simulink library "F3M_commonLib"  (R2023b)
settings: Solver=VariableStepAuto  StartTime=0.0  StopTime=10.0  RelTol=1e-3
undefined symbols (not defined in the file): entity, F3_getArrayPos, F3_getLossFilter, F3_ptableToArray, F3_ptableToGain, getIsoVec, isoelestring, m, n, Periodicity, pulsewidth, readAttrib, ressize, updateCurrentEProperties, updateInv
libraries: $bdroot x5
(part 1 of 2)
settings Model: Creator=nshoman  LastModifiedBy=nshoman

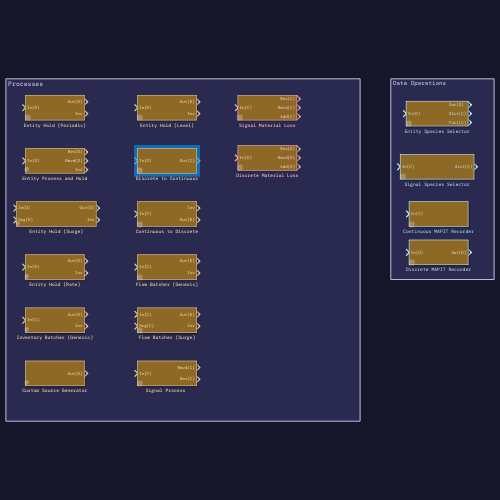
[thumbnail: Simulink's stored preview of the top-level diagram]
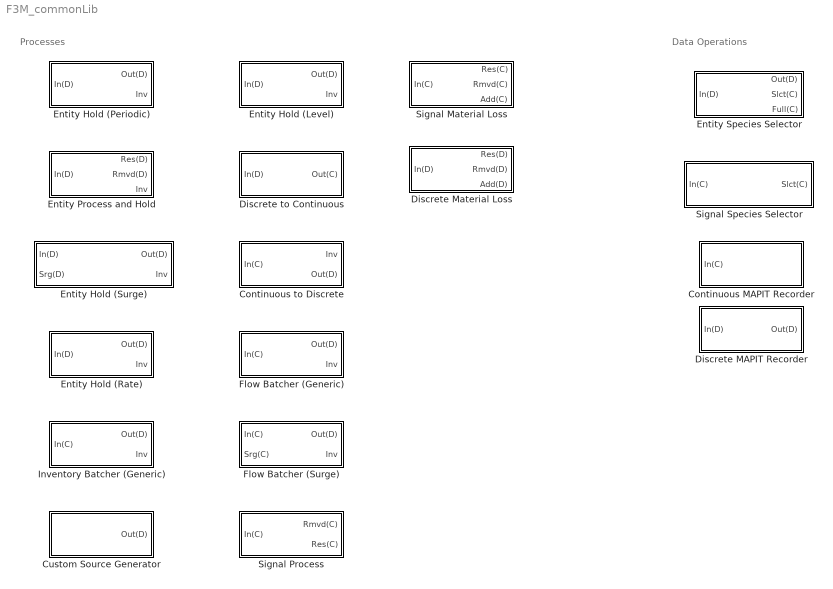
== system F3M_commonLib ==
  note: Processes
  note: Data Operations
  Continuous MAPIT Recorder : Subsystem  mask(Continuous MAPIT Recorder){wsname=simout1}
      mask prompts: wsname "Output variable name"
      mask help: F3M has been designed to work with MAPIT for downstream safeguards analyses. For a traditional material balance evaluation, flows must be integrated over the material balance period. It is important that data in F3M is collected so that, when integrated, input and output terms for the material balance is correct. Sampling too infrequently compared to the flow signals can result in pulses of material that are not recorded or truncated. However, high sampling rates can create excessively large datasets. This block balances these constraints by recording data with an inherited sample rate equal to the models major step, when the signal is non-zero. If the signal is zero, then information is not recorded
      mask init:
      | wsn = get_param(gcb,'wsname');
      |     set_param([gcb,'/TSS/MAPIT_OUT'],'VariableName',wsn);
      mask TypeOptions wsname: simout1
  Continuous to Discrete : Subsystem  mask(Continuous to Discrete){isoelestring=h, pulsewidth=1, size=10, ressize=0}
      mask prompts: isoelestring "Element or isotope (ex: h, u238)"; pulsewidth "Inventory pulse width (hr)"; size "Batch threshold (kg)"; ressize "Residual size (kg)"
      mask help: The continuous to discrete block converts a continuous Simulink signal into a discrete entity.
      mask TypeOptions isoelestring: h
  Custom Source Generator : Subsystem  mask(Custom Source Generator){size=10, period=5, ptable={'h3','1'}}
      mask prompts: size "Item size (kg)"; period "Item period (hr)"; ptable "Source specification table"
      mask help: The custom source generator is a template block for creating entity sources in F3M. The user must either define a source through the mask dialog options or create a function to do so. This block expects that sources will be specified in terms of weight percent expressed as a decimal. The block generates an entitiy with two different attributes, isovec and auxparams.
      mask DialogControl add_entry Prompt: Add entry
      mask DialogControl add_entry Callback:
      | maskObj = Simulink.Mask.get(gcb);
      |     tableControl = maskObj.getDialogControl('ptable');
      |     tableControl.addRow('a','b')
      mask DialogControl remove_entry Prompt: Remove entry
      mask DialogControl remove_entry Callback:
      | maskObj = Simulink.Mask.get(gcb);
      |     tableControl = maskObj.getDialogControl('ptable');
      |     nrow = tableControl.getNumberOfRows();
      |     if nrow>0
      |         tableControl.removeRow(nrow);
      |     end
  Discrete MAPIT Recorder : Subsystem  mask(Discrete MAPIT Recorder){InString=h, wsname=simout1}
      mask prompts: InString "Element or isotope (ex: h, u238)"; wsname "Output variable name"
      mask help: F3M has been designed to work with MAPIT for downstream safeguards analyses. For a traditional material balance evaluation, flows must be integrated over the material balance period. It is important that data in F3M is collected so that, when integrated, input and output terms for the material balance is correct. Discrete items simply output their entity attribute value when present, which eliminates the need for internal logic regarding sample frequency and searching for non-zero signals.
      mask init:
      | wsn = get_param(gcb,'wsname');
      |     set_param([gcb,'/TSS/MAPIT_OUT'],'VariableName',wsn);
      |     set_param([gcb,'/TSS1/MAPIT_OUT'],'VariableName',wsn);
      | 
      |     isn = get_param(gcb, 'InString');
      |     if strcmp(isn, 'all')
      |         set_param([gcb, '/TSS'], 'Commented', 'on');
      |         set_param([gcb, '/TSS1'], 'Commented', 'off');
      |     else
      |         set_param([gcb, '/TSS'], 'Commented', 'off');
      |         set_param([gcb, '/TSS1'], 'Commented', 'on');
      |     end
      mask TypeOptions InString: h
      mask TypeOptions wsname: simout1
  Discrete Material Loss : Subsystem  mask(Entity Material Loss){tStart=0, tEnd=0, lossFrac=0, lossOverride=off, lossOverrideTab={}, replaceBool=off, replaceTable={}}
      mask prompts: tStart "Start time (hr)"; tEnd "End time (hr)"; lossFrac "Removal fraction"; lossOverride "Loss species override"; replaceBool "Replacement material"
      mask help: The entity material loss block is designed to simulate loss, and optionally partial simultaneous replacement, of entities that enter the block. By default, the block removes a fraction of the entities entering the block during the specified interval. This behavior can be modified via the loss species override table wherein fractions can be set for individual elements or isotopes. A replacement table is available to specify replace lost material with a specified element or isotope with a certain fraction.
      mask init:
      | set_param(gcb,'MaskEnables',{'on';'on';'on';'on';'on';'on';'on'})
      |     maskObj = Simulink.Mask.get(gcb); 
      |     btnControl = maskObj.getDialogControl('addSub');
      |     btnControl.Enabled = "off";
      |     btnControl = maskObj.getDialogControl('removeSub');
      |     btnControl.Enabled = "off";
      |     btnControl = maskObj.getDialogControl('addLO');
      |     btnControl.Enabled = "off";
      |     btnControl = maskObj.getDialogControl('removeLO');
      |     btnControl.Enabled = "off";
      mask Callback lossOverride:
      | maskStr = get_param(gcb,'lossOverride');
      |     maskObj = Simulink.Mask.get(gcb);
      |     if strcmp(maskStr,'off')
      |        F = get_param(gcb,'MaskEnables');
      |        F{5} = 'off';
      |        set_param(gcb,'MaskEnables',F);
      |        btnControl = maskObj.getDialogControl('addLO');
      |        btnControl.Enabled = "off";
      |        btnControl = maskObj.getDialogControl('removeLO');
      |        btnControl.Enabled = "off";
      |     else
      |        F = get_param(gcb,'MaskEnables');
      |        F{5} = 'on';
      |        set_param(gcb,'MaskEnables',F);
      |        btnControl = maskObj.getDialogControl('addLO');
      |        btnControl.Enabled = "on";
      |        btnControl = maskObj.getDialogControl('removeLO');
      |        btnControl.Enabled = "on";
      |     end
      mask Callback replaceBool:
      | maskStr = get_param(gcb,'replaceBool');
      |     maskObj = Simulink.Mask.get(gcb);
      |     if strcmp(maskStr,'off')
      |        F = get_param(gcb,'MaskEnables');
      |        F{7} = 'off';
      |        set_param(gcb,'MaskEnables',F);
      |        btnControl = maskObj.getDialogControl('addSub');
      |        btnControl.Enabled = "off";
      |        btnControl = maskObj.getDialogControl('removeSub');
      |        btnControl.Enabled = "off";
      |     else
      |        F = get_param(gcb,'MaskEnables');
      |        F{7} = 'on';
      |        set_param(gcb,'MaskEnables',F);
      |        btnControl = maskObj.getDialogControl('addSub');
      |        btnControl.Enabled = "on";
      |        btnControl = maskObj.getDialogControl('removeSub');
      |        btnControl.Enabled = "on";
      |     end
      mask DialogControl addLO Prompt: Add
      mask DialogControl addLO Callback:
      | maskObj = Simulink.Mask.get(gcb);
      |     tableControl = maskObj.getDialogControl('lossOverrideTab');
      |     tableControl.addRow('a','b')
      mask DialogControl removeLO Prompt: Remove
      mask DialogControl removeLO Callback:
      | maskObj = Simulink.Mask.get(gcb);
      |     tableControl = maskObj.getDialogControl('lossOverrideTab');
      |     nrow = tableControl.getNumberOfRows();
      |     if nrow>0
      |         tableControl.removeRow(nrow);
      |     end
      mask DialogControl addSub Prompt: Add
      mask DialogControl addSub Callback:
      | maskObj = Simulink.Mask.get(gcb);
      |     tableControl = maskObj.getDialogControl('replaceTable');
      |     tableControl.addRow('a','b')
      mask DialogControl removeSub Prompt: Remove
      mask DialogControl removeSub Callback:
      | maskObj = Simulink.Mask.get(gcb);
      |     tableControl = maskObj.getDialogControl('replaceTable');
      |     nrow = tableControl.getNumberOfRows();
      |     if nrow>0
      |         tableControl.removeRow(nrow);
      |     end
  Discrete to Continuous : Subsystem  mask(Discrete to Continuous){width=eps}
      mask prompts: width "Pulse width"
      mask help: The discrete to continuous block converts a discrete entity into a continuous Simulink signal. The discrete item is represented by a square pulse with a width specified by the user. F3M will automatically scale the signal height such that the signal will integrate to the same elemental and isotopic values as the original entity.
      mask init:
      | mask_parameters = Simulink.Mask.get(gcb);
      | width_value = '';
      | for i = 1:length(mask_parameters.Parameters)
      |     if strcmp(mask_parameters.Parameters(i).Name, 'width')
      |         width_value = mask_parameters.Parameters(i).Value;
      |         break;
      |     end
      | end    
      | if strcmp(width_value, "eps")
      |     %width_internal = str2double(get_param(bdroot(),'MaxStep'));
      |     width_internal= 0.05;
      | else
      |     width_internal = str2double(width_value);
      | end
      mask Callback width:
      | mask_parameters = Simulink.Mask.get(gcb);
      | width_value = '';
      | for i = 1:length(mask_parameters.Parameters)
      |     if strcmp(mask_parameters.Parameters(i).Name, 'width')
      |         width_value = mask_parameters.Parameters(i).Value;
      |         break;
      |     end
      | end
      | if strcmp(width_value, "eps")
      |         %width_internal = str2double(get_param(bdroot(),'MaxStep'));
      |         width_internal = 0.05;
      | else
      |     width_internal = str2double(width_value);
      | end
  Entity Hold (Level) : Subsystem  mask(Entity Hold (Level)){nitems=0, time=0}
      mask prompts: nitems "Hold level (items)"; time "Process time (hr)"
      mask help: The entity hold (level) block simply holds a entities at a set level in a queue. If there are more items in queue than the level set point, then entities can leave the queue. The internal queue uses a First In First Out (FIFO) scheme. An optional process time is available which applies a time delay to an entity after it leaves the queue. This parameter can control how quickly entities are able to leave after the level set point has been reached. A continuous inventory term is updated whenever entities enter or leave the block.
  Entity Hold (Periodic) : Subsystem  mask(Entity Process and Hold){t_process=1}
      mask prompts: t_process "Process time (hr)"
      mask help: The entity hold (periodic) block simply holds an discrete entity for a period of time before releasing. The internal queue uses a First In First Out (FIFO) scheme. A continuous inventory term is updated whenever entities enter or leave the block.
  Entity Hold (Rate) : Subsystem  mask(Entity Hold (Rate)){rate=1}
      mask prompts: rate "Rate (item/hr)"
      mask help: This entity hold (rate) block simply holds a discrete entity in a queue. Entities are released at regular rate specified by the mask dialog parameters.
  Entity Hold (Surge) : Subsystem  mask(Entity Hold (Surge)){t_process=1}
      mask prompts: t_process "Process time"
      mask help: The entity hold (surge) block places input entities into a queue with a First In First Out (FIFO) scheme. Entities are only released when a surge signal is received.
  Entity Process and Hold : Subsystem  mask(Entity Process and Hold){t_process=1, ptable={'h3','0.10'}}
      mask prompts: t_process "Process time (hr)"
      mask help: The entity process and hold block holds a discrete entity for a period of time before releasing. If reduction multipliers are specified, then the entity is changed according to the reduction multipliers after any hold period has elapsed. The internal queue uses a First In First Out (FIFO) scheme. A continuous inventory term is updated when entities leave the queue.
      mask DialogControl addRowBtn Prompt: Add Entry
      mask DialogControl addRowBtn Callback:
      | maskObj = Simulink.Mask.get(gcb);
      |     tableControl = maskObj.getDialogControl('ptable');
      |     tableControl.addRow('a','b')
      mask DialogControl removeRowBtn Prompt: Remove Entry
      mask DialogControl removeRowBtn Callback:
      | maskObj = Simulink.Mask.get(gcb);
      |     tableControl = maskObj.getDialogControl('ptable');
      |     nrow = tableControl.getNumberOfRows();
      |     if nrow>0
      |         tableControl.removeRow(nrow);
      |     end
  Entity Species Selector : Subsystem  mask(Entity Species Selector){InString=h, width=0.10}
      mask prompts: InString "Element or isotope (ex: h, u238)"; width "Pulse width"
      mask help: The entity species selector extracts the specified isotope or element attributes of an entity (multiple if several isotopes for the element are tracked). The full signal is also returned, which can be combined with multiple signal selector blocks for additional species-specific signals if desired. This is a convenience block to select certain species of interest from the [1677, 1] shaped attribute that F3M uses for most modeling operations.
      mask TypeOptions InString: h
  Flow Batcher (Generic) : Subsystem  mask(Flow Batcher (Generic)){p1=h, p2=1, p3=0, p4=0}
      mask prompts: p1 "Batch basis (ex: h, u238)"; p2 "Inventory pulse width (hr)"; p3 "Output target size (kg)"; p4 "Residual size (kg)"
      mask help: The generic flow batcher creates discrete entities from an input flow according to user defined settings in the dialog (i.e., creates a batch). The generic flow batcher uses an isotope or element (or other keyword, see overview page) combined with a target size to create an entity.
      mask TypeOptions p1: h
  Flow Batcher (Surge) : Subsystem  mask(Flow Batcher (Surge)){isoelestring=h1, pulsewidth=0, size=0, ressize=0}
      mask prompts: isoelestring "Element or isotope (ex: h, u238)"; pulsewidth "Pulse width (hr)"; size "Output target size (kg)"; ressize "Residual size (kg)"
      mask help: The surge flow batcher creates discrete entities from an input flow according to user defined settings in the dialog (i.e., creates a batch). The surge flow batcher uses an isotope or element (or other keyword, see overview page) combined with a target size to create an entity when a surge signal is supplied.
      mask TypeOptions isoelestring: h1
  Inventory Batcher (Generic) : Subsystem  mask(Inventory Batcher (Generic)){p1=h, p2=1, p3=0, p4=0}
      mask prompts: p1 "Batch basis (ex: h, u238)"; p2 "Inventory pulse width (hr)"; p3 "Output target size (kg)"; p4 "Residual size (kg)"
      mask help: The generic inventory batcher creates discrete entities from an input flow according to user defined settings in the dialog (i.e., creates a batch). This block is similar to the generic flow batcher with the key difference that this block will not output while flow is entering. It is designed to be used with inventories, rather than flows, and expects that there will be periodic, rather than continuous, additions to the inventory will be made.
      mask TypeOptions p1: h
  Signal Material Loss : Subsystem  mask(Signal Material Loss){tStart=0, tEnd=0, lossFrac=0, lossOverride=off, lossOverrideTab={}, replaceBool=off, replaceTable={}}
      mask prompts: tStart "Start time (hr)"; tEnd "End time (hr)"; lossFrac "Removal fraction"; lossOverride "Loss species override"; replaceBool "Replacement material"
      mask help: The signal material loss block is designed to simulate material loss, and optionally simultaneous replacement, of material stream represented by a signal. By default, the block removes a fraction of the signal for the specified amount of time. This behavior can be modified via the loss species override table wherein fractions can be set for individual elements or isotopes. A replacement table is available to specify replace lost material with a specified element or isotope with a certain fraction.
      mask init:
      | set_param(gcb,'MaskEnables',{'on';'on';'on';'on';'on';'on';'on'})
      |     maskObj = Simulink.Mask.get(gcb); 
      |     btnControl = maskObj.getDialogControl('addSub');
      |     btnControl.Enabled = "off";
      |     btnControl = maskObj.getDialogControl('removeSub');
      |     btnControl.Enabled = "off";
      |     btnControl = maskObj.getDialogControl('addLO');
      |     btnControl.Enabled = "off";
      |     btnControl = maskObj.getDialogControl('removeLO');
      |     btnControl.Enabled = "off";
      mask Callback lossOverride:
      | maskStr = get_param(gcb,'lossOverride');
      |     maskObj = Simulink.Mask.get(gcb);
      |     if strcmp(maskStr,'off')
      |        F = get_param(gcb,'MaskEnables');
      |        F{5} = 'off';
      |        set_param(gcb,'MaskEnables',F);
      |        btnControl = maskObj.getDialogControl('addLO');
      |        btnControl.Enabled = "off";
      |        btnControl = maskObj.getDialogControl('removeLO');
      |        btnControl.Enabled = "off";
      |     else
      |        F = get_param(gcb,'MaskEnables');
      |        F{5} = 'on';
      |        set_param(gcb,'MaskEnables',F);
      |        btnControl = maskObj.getDialogControl('addLO');
      |        btnControl.Enabled = "on";
      |        btnControl = maskObj.getDialogControl('removeLO');
      |        btnControl.Enabled = "on";
      |     end
      mask Callback replaceBool:
      | maskStr = get_param(gcb,'replaceBool');
      |     maskObj = Simulink.Mask.get(gcb);
      |     if strcmp(maskStr,'off')
      |        F = get_param(gcb,'MaskEnables');
      |        F{7} = 'off';
      |        set_param(gcb,'MaskEnables',F);
      |        btnControl = maskObj.getDialogControl('addSub');
      |        btnControl.Enabled = "off";
      |        btnControl = maskObj.getDialogControl('removeSub');
      |        btnControl.Enabled = "off";
      |     else
      |        F = get_param(gcb,'MaskEnables');
      |        F{7} = 'on';
      |        set_param(gcb,'MaskEnables',F);
      |        btnControl = maskObj.getDialogControl('addSub');
      |        btnControl.Enabled = "on";
      |        btnControl = maskObj.getDialogControl('removeSub');
      |        btnControl.Enabled = "on";
      |     end
      mask DialogControl addLO Prompt: Add
      mask DialogControl addLO Callback:
      | maskObj = Simulink.Mask.get(gcb);
      |     tableControl = maskObj.getDialogControl('lossOverrideTab');
      |     tableControl.addRow('a','b')
      mask DialogControl removeLO Prompt: Remove
      mask DialogControl removeLO Callback:
      | maskObj = Simulink.Mask.get(gcb);
      |     tableControl = maskObj.getDialogControl('lossOverrideTab');
      |     nrow = tableControl.getNumberOfRows();
      |     if nrow>0
      |         tableControl.removeRow(nrow);
      |     end
      mask DialogControl addSub Prompt: Add
      mask DialogControl addSub Callback:
      | maskObj = Simulink.Mask.get(gcb);
      |     tableControl = maskObj.getDialogControl('replaceTable');
      |     tableControl.addRow('a','b')
      mask DialogControl removeSub Prompt: Remove
      mask DialogControl removeSub Callback:
      | maskObj = Simulink.Mask.get(gcb);
      |     tableControl = maskObj.getDialogControl('replaceTable');
      |     nrow = tableControl.getNumberOfRows();
      |     if nrow>0
      |         tableControl.removeRow(nrow);
      |     end
  "Signal Process " : Subsystem  mask(Signal Process){ptable={}}
      mask help: The signal process block applies user specified modification fractions to the signal to simulate a process. These values are assumed to be in [0,1], although any float can be provided.
      mask DialogControl addRowBtn Prompt: Add Entry
      mask DialogControl addRowBtn Callback:
      | maskObj = Simulink.Mask.get(gcb);
      |     tableControl = maskObj.getDialogControl('ptable');
      |     tableControl.addRow('a','b')
      mask DialogControl removeRowBtn Prompt: Remove Entry
      mask DialogControl removeRowBtn Callback:
      | maskObj = Simulink.Mask.get(gcb);
      |     tableControl = maskObj.getDialogControl('ptable');
      |     nrow = tableControl.getNumberOfRows();
      |     if nrow>0
      |         tableControl.removeRow(nrow);
      |     end
  Signal Species Selector : Subsystem  mask(Signal Species Selector){InString=h}
      mask prompts: InString "Element or isotope (ex: h, u238)"
      mask help: The signal species selector extracts the specified isotope signal or element signal (multiple if several isotopes for the element are tracked). This is a convenience block to select certain species of interest from the [1677, 1] shaped signal that F3M uses for most modeling operations.
      mask TypeOptions InString: h

== system F3M_commonLib/Continuous MAPIT Recorder ==
  In(C) : Inport
  Constant : Constant
  Constant1 : Constant  Value=0
  Memory : Memory
  Memory1 : Memory
  Memory2 : Memory
  Sum : Sum  Inputs=++++
  Sum of Elements : Sum  Inputs=+
  Switch : Switch  Criteria=u2 ~= 0  SaturateOnIntegerOverflow=off  InputSameDT=off
  TSS : Subsystem  TreatAsAtomicUnit=on
  wires:
  Constant/1 -> Switch/1
  Constant1/1 -> Switch/3
  In(C)/1 -> TSS/1(In(C)), Sum of Elements/1
  Sum of Elements/1 -> Switch/2
  Switch/1 -> Sum/1, Memory/1
  Memory/1 -> Sum/2, Memory1/1
  Memory1/1 -> Sum/3, Memory2/1
  Sum/1 -> TSS/Enable
  Memory2/1 -> Sum/4

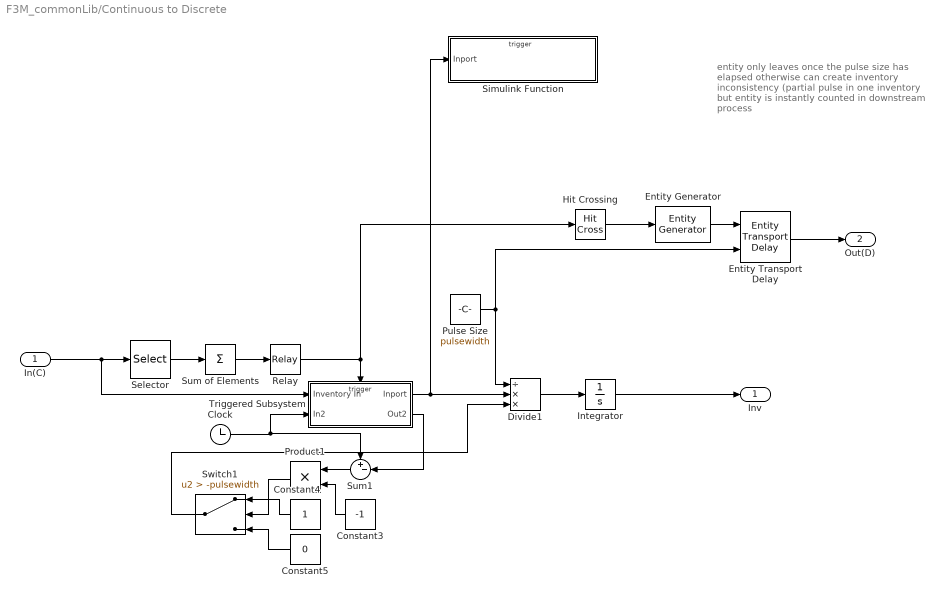
== system F3M_commonLib/Continuous to Discrete ==
  note: entity only leaves once
      | the pulse size has elapsed
      | otherwise can create inventory
      | inconsistency (partial pulse
      | in one inventory but entity is
      | instantly counted in downstream
      | process
  In(C) : Inport
  Clock : Clock
  Constant3 : Constant  Value=-1
  Constant4 : Constant
  Constant5 : Constant  Value=0
  Divide1 : Product  Inputs=/**
  Entity Transport Delay : EntityTransportDelay  InputPortMessageModes=m,n  OutputPortMessageModes=m
  Entity Generator : EntityGenerator  InputPortMessageModes=m  OutputPortMessageModes=m  GenerationMethod=Event-based  GenerateAction=entity.isovec = updateIsovec();  AttributeName=isovec|auxparam  AttributeInitialValue=zeros(1677,1)|1  EntityType=Structured  EntityTypeName=Entity
      settings: InputPortMap=u0
  Hit Crossing : HitCross  OutputPortMessageModes=m  HitCrossingOffset=1  HitCrossingDirection=rising  HitCrossingOutputType=Message
  Integrator : Integrator
  Product1 : Product
  Pulse Size : Constant  Value=pulsewidth
  Relay : Relay  OnSwitchValue=size  OffSwitchValue=ressize
  Selector : Selector  InputPortWidth=1677  IndexOptions=Index vector (dialog)  Indices=F3_getArrayPos(isoelestring)  OutputSizes=1
  Simulink Function : Subsystem  TreatAsAtomicUnit=on
  Sum of Elements : Sum  Inputs=+
  Sum1 : Sum  Inputs=+-|
  Switch1 : Switch  Criteria=u2 > Threshold  Threshold=-pulsewidth  SaturateOnIntegerOverflow=off  InputSameDT=off
      settings: AttributesFormatString=-pulseSize
  Triggered Subsystem : Subsystem  TreatAsAtomicUnit=on
  Inv : Outport
  Out(D) : Outport  Port=2
  wires:
  Integrator/1 -> Inv/1
  Clock/1 -> Sum1/1, Triggered Subsystem/2(In2)
  Constant5/1 -> Switch1/3
  Sum of Elements/1 -> Relay/1
  Constant3/1 -> Product1/2
  Relay/1 -> Hit Crossing/1, Triggered Subsystem/Trigger
  Triggered Subsystem/2(Out2) -> Sum1/2
  Divide1/1 -> Integrator/1
  Switch1/1 -> Divide1/3
  Triggered Subsystem/1(Inport) -> Divide1/2, Simulink Function/1(Inport)
  In(C)/1 -> Triggered Subsystem/1(Inventory In), Selector/1
  Product1/1 -> Switch1/2
  Constant4/1 -> Switch1/1
  Sum1/1 -> Product1/1
  Selector/1 -> Sum of Elements/1
  Hit Crossing/1 -> Entity Generator/1
  Entity Generator/1 -> Entity Transport Delay/1
  Entity Transport Delay/1 -> Out(D)/1
  Pulse Size/1 -> Entity Transport Delay/2, Divide1/1

== system F3M_commonLib/Custom Source Generator ==
  Entity Generator : EntityGenerator  OutputPortMessageModes=m  Period=period  GenerateAction=entity.isovec = getInitialIsos();  AttributeName=isovec|auxparam  AttributeInitialValue=zeros(1677,1)|1  EntityType=Structured  EntityTypeName=Entity
  Simulink Function : Subsystem  TreatAsAtomicUnit=on
  Out(D) : Outport
  wires:
  Entity Generator/1 -> Out(D)/1

== system F3M_commonLib/Discrete MAPIT Recorder ==
  In(D) : Inport
  Entity Server : EntityServer  InputPortMessageModes=m  OutputPortMessageModes=m  Capacity=1  ServiceTimeValue=0  ExitAction=readAttrib(entity.isovec)
  TSS : Subsystem  TreatAsAtomicUnit=on
  TSS1 : Subsystem  Commented=on  TreatAsAtomicUnit=on
  Out(D) : Outport
  wires:
  In(D)/1 -> Entity Server/1
  Entity Server/1 -> Out(D)/1

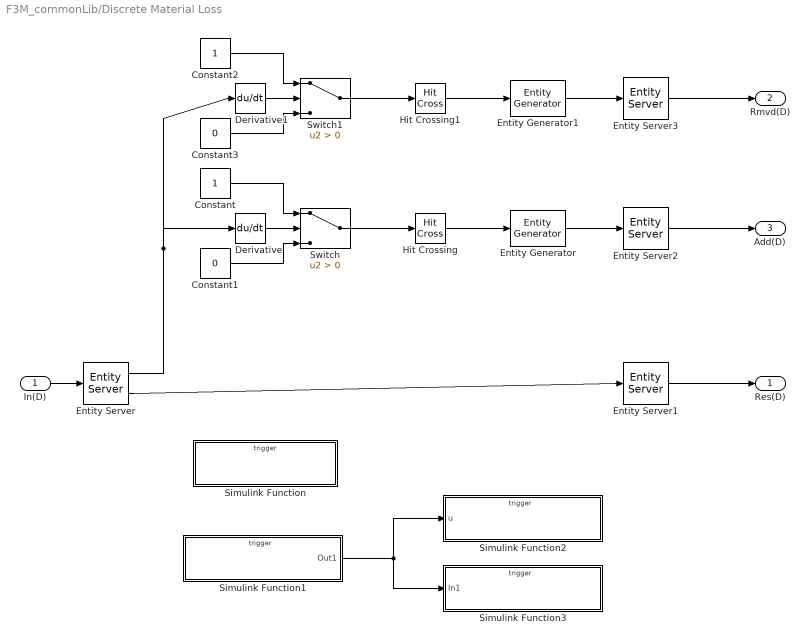
== system F3M_commonLib/Discrete Material Loss ==
  In(D) : Inport
  Constant : Constant
  Constant1 : Constant  Value=0
  Constant2 : Constant
  Constant3 : Constant  Value=0
  Derivative : Derivative
  Derivative1 : Derivative
  Entity Generator : EntityGenerator  InputPortMessageModes=m  OutputPortMessageModes=m  GenerationMethod=Event-based  AttributeName=isovec|auxparam  AttributeInitialValue=zeros(1677,1)|1  EntityType=Structured  EntityTypeName=Entity
      settings: InputPortMap=u0
  Entity Generator1 : EntityGenerator  InputPortMessageModes=m  OutputPortMessageModes=m  GenerationMethod=Event-based  AttributeName=isovec|auxparam  AttributeInitialValue=zeros(1677,1)|1  EntityType=Structured  EntityTypeName=Entity
      settings: InputPortMap=u0
  Entity Server : EntityServer  InputPortMessageModes=m  OutputPortMessageModes=n,m  Capacity=inf  ServiceTimeValue=0  EntryAction=updateCurrentEProperties(entity.isovec);  NumberEntitiesDeparted=on
      settings: OutputPortMap=o0,o9
  Entity Server1 : EntityServer  InputPortMessageModes=m  OutputPortMessageModes=m  Capacity=inf  ServiceTimeValue=0  ServiceCompleteAction=entity.isovec = applyAllFilters(entity.isovec);
  Entity Server2 : EntityServer  InputPortMessageModes=m  OutputPortMessageModes=m  Capacity=inf  ServiceTimeValue=0  ServiceCompleteAction=entity.isovec=applyGainFilterGainE();
  Entity Server3 : EntityServer  InputPortMessageModes=m  OutputPortMessageModes=m  Capacity=inf  ServiceTimeValue=0  ServiceCompleteAction=entity.isovec=applyLossFilterLossE();
  Hit Crossing : HitCross  HitCrossingDirection=rising  HitCrossingOutputType=Message
  Hit Crossing1 : HitCross  HitCrossingDirection=rising  HitCrossingOutputType=Message
  Simulink Function : Subsystem  TreatAsAtomicUnit=on
  Simulink Function1 : Subsystem  TreatAsAtomicUnit=on
  Simulink Function2 : Subsystem  TreatAsAtomicUnit=on
  Simulink Function3 : Subsystem  TreatAsAtomicUnit=on
  Switch : Switch  Criteria=u2 > Threshold  SaturateOnIntegerOverflow=off  InputSameDT=off
  Switch1 : Switch  Criteria=u2 > Threshold  SaturateOnIntegerOverflow=off  InputSameDT=off
  Res(D) : Outport
  Rmvd(D) : Outport  Port=2
  Add(D) : Outport  Port=3
  wires:
  In(D)/1 -> Entity Server/1
  Entity Server/2 -> Entity Server1/1
  Entity Server1/1 -> Res(D)/1
  Derivative/1 -> Switch/2
  Entity Server/1 -> Derivative1/1, Derivative/1
  Constant/1 -> Switch/1
  Constant1/1 -> Switch/3
  Switch/1 -> Hit Crossing/1
  Entity Generator/1 -> Entity Server2/1
  Entity Server2/1 -> Add(D)/1
  Hit Crossing/1 -> Entity Generator/1
  Entity Server3/1 -> Rmvd(D)/1
  Entity Generator1/1 -> Entity Server3/1
  Constant2/1 -> Switch1/1
  Switch1/1 -> Hit Crossing1/1
  Constant3/1 -> Switch1/3
  Hit Crossing1/1 -> Entity Generator1/1
  Derivative1/1 -> Switch1/2
  Simulink Function1/1(Out1) -> Simulink Function3/1(In1), Simulink Function2/1(u)

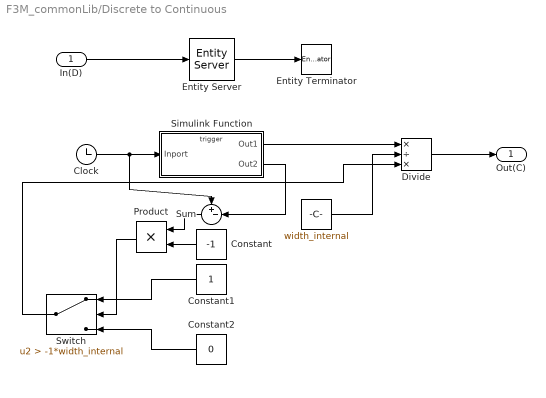
== system F3M_commonLib/Discrete to Continuous ==
  In(D) : Inport
  " " : Constant  Value=width_internal
  Clock : Clock
  Constant : Constant  Value=-1
  Constant1 : Constant
  Constant2 : Constant  Value=0
  Divide : Product  Inputs=*/*
  Entity Server : EntityServer  InputPortMessageModes=m  OutputPortMessageModes=m  Capacity=1  ExitAction=getIsoVec(entity.isovec);
  Entity Terminator : EntityTerminator  InputPortMessageModes=m
  Product : Product
  Simulink Function : Subsystem  TreatAsAtomicUnit=on
  Sum : Sum  Inputs=+-|
  Switch : Switch  Criteria=u2 > Threshold  Threshold=-1*width_internal  SaturateOnIntegerOverflow=off  InputSameDT=off
  Out(C) : Outport
  wires:
  In(D)/1 -> Entity Server/1
  Entity Server/1 -> Entity Terminator/1
  Clock/1 -> Sum/1, Simulink Function/1(Inport)
  Simulink Function/1(Out1) -> Divide/1
  Divide/1 -> Out(C)/1
  Simulink Function/2(Out2) -> Sum/2
  Sum/1 -> Product/1
  Constant/1 -> Product/2
  Constant2/1 -> Switch/3
  Constant1/1 -> Switch/1
  Product/1 -> Switch/2
  Switch/1 -> Divide/3
  " "/1 -> Divide/2

== system F3M_commonLib/Entity Hold (Level) ==
  In(D) : Inport
  Constant : Constant
  Constant1 : Constant  Value=-1
  Entity Gate : EntityGate  InputPortMessageModes=m,m  OutputPortMessageModes=m
  Entity Server : EntityServer  InputPortMessageModes=m  OutputPortMessageModes=n,m  Capacity=inf  ServiceTimeValue=0  EntryAction=updateInv(entity.isovec,1)  NumberEntitiesInBlock=on
      settings: OutputPortMap=o1,o9
  Entity Server1 : EntityServer  InputPortMessageModes=m  OutputPortMessageModes=m  Capacity=1  ServiceTimeValue=time  ExitAction=updateInv(entity.isovec,-1)
  Message Send : Send  OutputPortMessageModes=m
  Simulink Function1 : $bdroot/Entity Hold (Periodic)/Simulink Function  SystemSampleTime=-1  VariantActivationTime=update diagram  AllowFlexibleInterface=on  Latency=0  AutoFrameSizeCalculation=off
      settings: LibrarySourceBlock=sldelib/Simulink Function
  Switch : Switch  Threshold=nitems  SaturateOnIntegerOverflow=off  InputSameDT=off
  Out(D) : Outport
  Inv : Outport  Port=2
  wires:
  Simulink Function1/1 -> Inv/1
  In(D)/1 -> Entity Server/1
  Entity Server/2 -> Entity Gate/2
  Entity Gate/1 -> Entity Server1/1
  Entity Server1/1 -> Out(D)/1
  Entity Server/1 -> Switch/2
  Constant/1 -> Switch/1
  Constant1/1 -> Switch/3
  Switch/1 -> Message Send/1
  Message Send/1 -> Entity Gate/1

== system F3M_commonLib/Entity Hold (Periodic) ==
  "In(D) " : Inport
  Entity Server1 : EntityServer  InputPortMessageModes=m  OutputPortMessageModes=m  Capacity=inf  ServiceTimeValue=t_process  EntryAction=updateInv(entity.isovec,1)  ExitAction=updateInv(entity.isovec,-1)
  Simulink Function : Subsystem  TreatAsAtomicUnit=on
      settings: LibrarySourceBlock=sldelib/Simulink Function
  Out(D) : Outport
  Inv : Outport  Port=2
  wires:
  "In(D) "/1 -> Entity Server1/1
  Entity Server1/1 -> Out(D)/1
  Simulink Function/1(y) -> Inv/1

== system F3M_commonLib/Entity Hold (Rate) ==
  In(D) : Inport
  Entity Server : EntityServer  InputPortMessageModes=m  OutputPortMessageModes=m  Capacity=inf  ServiceTimeValue=1/rate
  Simulink Function : $bdroot/Entity Hold (Periodic)/Simulink Function  SystemSampleTime=-1  VariantActivationTime=update diagram  AllowFlexibleInterface=on  Latency=0  AutoFrameSizeCalculation=off
      settings: LibrarySourceBlock=sldelib/Simulink Function
  Out(D) : Outport
  Inv : Outport  Port=2
  wires:
  In(D)/1 -> Entity Server/1
  Entity Server/1 -> Out(D)/1
  Simulink Function/1 -> Inv/1

== system F3M_commonLib/Entity Hold (Surge) ==
  In(D) : Inport
  Srg(D) : Inport  Port=2
  Entity Gate : EntityGate  InputPortMessageModes=m,m  OutputPortMessageModes=m
  Entity Queue : Queue  InputPortMessageModes=m  OutputPortMessageModes=m  Capacity=inf
  Entity Server : EntityServer  InputPortMessageModes=m  OutputPortMessageModes=m  Capacity=inf  ServiceTimeValue=t_process  EntryAction=updateInv(entity.isovec,1)
  Entity Server1 : EntityServer  InputPortMessageModes=m  OutputPortMessageModes=m  Capacity=inf  ServiceTimeValue=0  ExitAction=updateInv(entity.isovec,-1)
  Simulink Function1 : $bdroot/Entity Hold (Periodic)/Simulink Function  SystemSampleTime=-1  VariantActivationTime=update diagram  AllowFlexibleInterface=on  Latency=0  AutoFrameSizeCalculation=off
      settings: LibrarySourceBlock=sldelib/Simulink Function
  Out(D) : Outport
  Inv : Outport  Port=2
  wires:
  Entity Queue/1 -> Entity Gate/2
  Entity Gate/1 -> Entity Server1/1
  Srg(D)/1 -> Entity Gate/1
  In(D)/1 -> Entity Server/1
  Entity Server/1 -> Entity Queue/1
  Entity Server1/1 -> Out(D)/1
  Simulink Function1/1 -> Inv/1

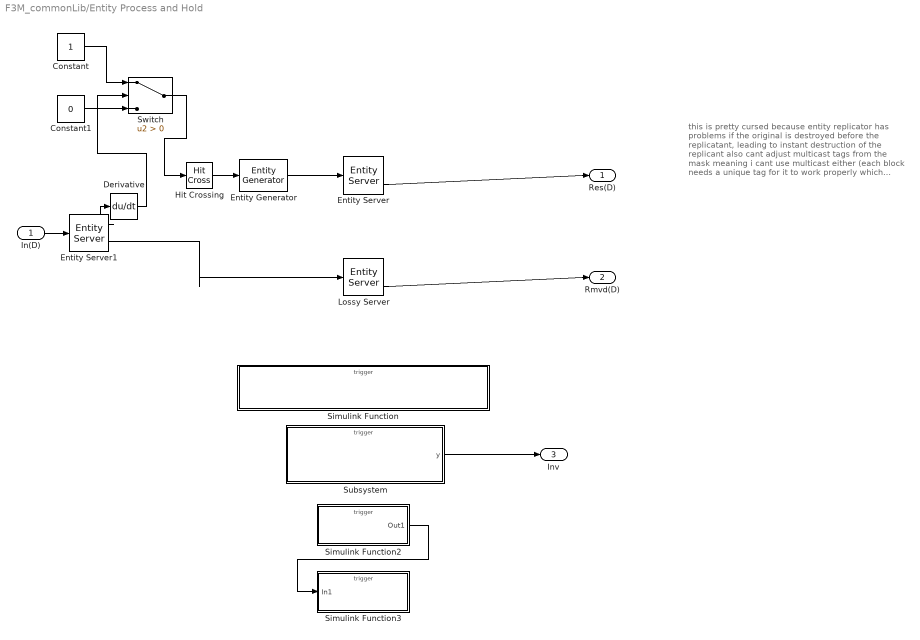
== system F3M_commonLib/Entity Process and Hold ==
  note: this is pretty cursed because
      | entity replicator has problems
      | if the original is destroyed
      | before the replicatant, leading
      | to instant destruction of the
      | replicant
      |
      | also cant adjust multicast tags
      | from the mask meaning i cant
      | use multicast either (each
      | block needs a unique tag
      | for it to work properly which
      | needs to be assigned programatically)
      |
      | the multiple servers ensures
      | things happen in the proper order
  In(D) : Inport
  Constant : Constant
  Constant1 : Constant  Value=0
  Derivative : Derivative
  Entity Generator : EntityGenerator  InputPortMessageModes=m  OutputPortMessageModes=m  GenerationMethod=Event-based  Period=Periodicity  GenerateAction=entity.isovec = getEntityValue();  AttributeName=isovec|auxparam  AttributeInitialValue=zeros(1677,1)|1  EntityType=Structured  EntityTypeName=Entity
      settings: InputPortMap=u0
  Entity Server : EntityServer  InputPortMessageModes=m  OutputPortMessageModes=n,m  Capacity=inf  ServiceTimeValue=t_process  ServiceCompleteAction=entity.isovec=calculateNewEntity(entity.isovec,0);  ExitAction=updateInv(entity.isovec,-1)  NumberEntitiesDeparted=on
      settings: OutputPortMap=o0,o9
  Entity Server1 : EntityServer  InputPortMessageModes=m  OutputPortMessageModes=n,m  Capacity=inf  ServiceTimeValue=0  EntryAction=|  NumberEntitiesDeparted=on
      | updateInv(entity.isovec,1)
      | updateLatestEntity(entity.isovec);
      settings: OutputPortMap=o0,o9
  Hit Crossing : HitCross  OutputPortMessageModes=m  HitCrossingDirection=rising  HitCrossingOutputType=Message
  Lossy Server : EntityServer  InputPortMessageModes=m  OutputPortMessageModes=n,m  Capacity=inf  ServiceTimeValue=t_process  ServiceCompleteAction=entity.isovec=calculateNewEntity(entity.isovec,1);  ExitAction=updateInv(entity.isovec,-1)  NumberEntitiesDeparted=on
      settings: OutputPortMap=o0,o9
  Simulink Function : Subsystem  TreatAsAtomicUnit=on
      settings: LibrarySourceBlock=sldelib/Simulink Function
  Simulink Function2 : Subsystem  TreatAsAtomicUnit=on
  Simulink Function3 : Subsystem  TreatAsAtomicUnit=on
  Subsystem : Subsystem
  Switch : Switch  Criteria=u2 > Threshold  SaturateOnIntegerOverflow=off  InputSameDT=off
  Res(D) : Outport
  Rmvd(D) : Outport  Port=2
  Inv : Outport  Port=3
  wires:
  Hit Crossing/1 -> Entity Generator/1
  Entity Generator/1 -> Entity Server/1
  Lossy Server/2 -> Rmvd(D)/1
  Switch/1 -> Hit Crossing/1
  Entity Server/2 -> Res(D)/1
  Subsystem/1(y) -> Inv/1
  Entity Server1/2 -> Lossy Server/1
  Constant/1 -> Switch/1
  Simulink Function2/1(Out1) -> Simulink Function3/1(In1)
  Entity Server1/1 -> Derivative/1
  Constant1/1 -> Switch/3
  Derivative/1 -> Switch/2
  In(D)/1 -> Entity Server1/1

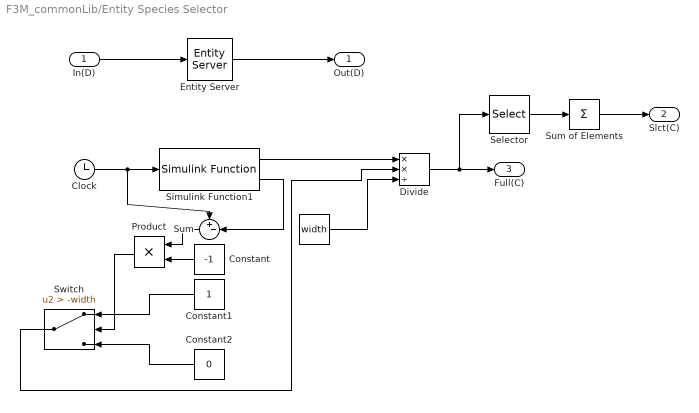
== system F3M_commonLib/Entity Species Selector ==
  In(D) : Inport
  " " : Constant  Value=width
  Clock : Clock
  Constant : Constant  Value=-1
  Constant1 : Constant
  Constant2 : Constant  Value=0
  Divide : Product  Inputs=**/
  Entity Server : EntityServer  InputPortMessageModes=m  OutputPortMessageModes=m  Capacity=inf  ServiceTimeValue=0  ExitAction=getIsoVec(entity.isovec)
  Product : Product
  Selector : Selector  InputPortWidth=1677  IndexOptions=Index vector (dialog)  Indices=F3_getArrayPos(InString)  OutputSizes=1
  Simulink Function1 : $bdroot/Discrete to Continuous/Simulink Function  SystemSampleTime=-1  VariantActivationTime=update diagram  AllowFlexibleInterface=on  Latency=0  AutoFrameSizeCalculation=off
  Sum : Sum  Inputs=+-|
  Sum of Elements : Sum  Inputs=+
  Switch : Switch  Criteria=u2 > Threshold  Threshold=-width  SaturateOnIntegerOverflow=off  InputSameDT=off
  "Out(D) " : Outport
  Slct(C) : Outport  Port=2
  Full(C) : Outport  Port=3
  wires:
  In(D)/1 -> Entity Server/1
  Entity Server/1 -> "Out(D) "/1
  Constant/1 -> Product/2
  Simulink Function1/1 -> Divide/1
  Constant2/1 -> Switch/3
  Sum/1 -> Product/1
  Divide/1 -> Selector/1, Full(C)/1
  Simulink Function1/2 -> Sum/2
  Clock/1 -> Sum/1, Simulink Function1/1
  Product/1 -> Switch/2
  Constant1/1 -> Switch/1
  " "/1 -> Divide/3
  Switch/1 -> Divide/2
  Selector/1 -> Sum of Elements/1
  Sum of Elements/1 -> Slct(C)/1

== system F3M_commonLib/Flow Batcher (Generic) ==
  In(C) : Inport
  "Continuous to Discrete " : Subsystem  Description=requires eval on mask so isn't a direct link of continuous to discrete  mask{isoelestring=p1, pulsewidth=p2, size=p3, ressize=p4}
      mask prompts: isoelestring "Element or isotope (ex: h, u238)"; pulsewidth "Pulse width (hr)"; size "Output target size (kg)"; ressize "Residual size (kg)"
      mask TypeOptions isoelestring: h
  Integrator : Integrator
  Sum : Sum  Inputs=+-
  Out(D) : Outport
  Inv : Outport  Port=2
  wires:
  In(C)/1 -> Integrator/1
  Integrator/1 -> Sum/1
  Sum/1 -> "Continuous to Discrete "/1(Inventory In), Inv/1
  "Continuous to Discrete "/2(Entity) -> Out(D)/1
  "Continuous to Discrete "/1(Inventory Reduce) -> Sum/2

== system F3M_commonLib/Flow Batcher (Surge) ==
  In(C) : Inport
  Srg(C) : Inport  Port=2
  Continuous to Discrete (Surge) : Subsystem  mask{isoelestring=isoelestring, pulsewidth=pulsewidth, size=size, ressize=ressize}
      mask prompts: isoelestring "Element or isotope (ex: h, u238)"; pulsewidth "Pulse width (hr)"; size "Output target size (kg)"; ressize "Residual size (kg)"
      mask TypeOptions isoelestring: isoelestring
  Integrator : Integrator
  Sum : Sum  Inputs=+-
  Out(D) : Outport
  Inv : Outport  Port=2
  wires:
  In(C)/1 -> Integrator/1
  Integrator/1 -> Sum/1
  Sum/1 -> Continuous to Discrete (Surge)/1(Inventory In), Inv/1
  Srg(C)/1 -> Continuous to Discrete (Surge)/2(Surge)
  Continuous to Discrete (Surge)/1(Inventory Reduce) -> Sum/2
  Continuous to Discrete (Surge)/2(Entity) -> Out(D)/1

== system F3M_commonLib/Inventory Batcher (Generic) ==
  In(C) : Inport
  Batcher : Subsystem
  Integrator : Integrator
  Sum : Sum  Inputs=+-
  Out(D) : Outport
  Inv : Outport  Port=2
  wires:
  In(C)/1 -> Integrator/1
  Integrator/1 -> Sum/1
  Sum/1 -> Batcher/1(Inventory In), Inv/1
  Batcher/1(Reduce) -> Sum/2
  Batcher/2(Entity) -> Out(D)/1

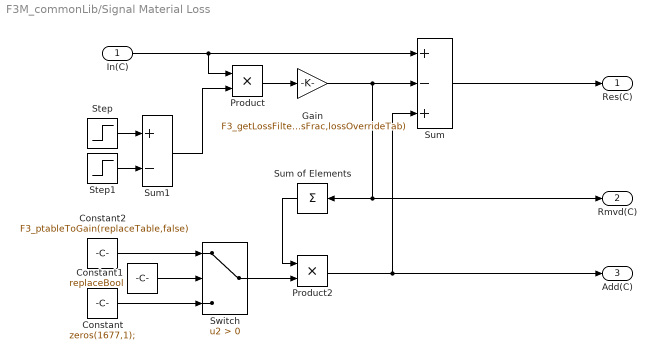
== system F3M_commonLib/Signal Material Loss ==
  In(C) : Inport
  Constant : Constant  Value=zeros(1677,1);
  Constant1 : Constant  Value=replaceBool
  Constant2 : Constant  Value=F3_ptableToGain(replaceTable,false)
  Gain : Gain  Gain=F3_getLossFilter(lossFrac,lossOverrideTab)
  Product : Product
  Product2 : Product
  Step : Step  Time=tStart  SampleTime=0
  Step1 : Step  Time=tEnd  SampleTime=0
  Sum : Sum  Inputs=+-+
  Sum of Elements : Sum  Inputs=+
  Sum1 : Sum  Inputs=+-
  Switch : Switch  Criteria=u2 > Threshold  SaturateOnIntegerOverflow=off  InputSameDT=off
  Res(C) : Outport
  Rmvd(C) : Outport  Port=2
  Add(C) : Outport  Port=3
  wires:
  Sum/1 -> Res(C)/1
  In(C)/1 -> Product/1, Sum/1
  Product/1 -> Gain/1
  Step/1 -> Sum1/1
  Step1/1 -> Sum1/2
  Sum1/1 -> Product/2
  Gain/1 -> Rmvd(C)/1, Sum of Elements/1, Sum/2
  Switch/1 -> Product2/2
  Constant/1 -> Switch/3
  Constant1/1 -> Switch/2
  Constant2/1 -> Switch/1
  Sum of Elements/1 -> Product2/1
  Product2/1 -> Sum/3, Add(C)/1

== system F3M_commonLib/Signal Process  ==
  In(C) : Inport
  Gain : Gain  Gain=F3_ptableToGain(ptable,false)
  Sum : Sum  Inputs=-+|
  Rmvd(C) : Outport
  Res(C) : Outport  Port=2
  wires:
  In(C)/1 -> Sum/2, Gain/1
  Gain/1 -> Rmvd(C)/1, Sum/1
  Sum/1 -> Res(C)/1

== system F3M_commonLib/Signal Species Selector ==
  In(C) : Inport
  Selector : Selector  InputPortWidth=1677  IndexOptions=Index vector (dialog)  Indices=F3_getArrayPos(InString)  OutputSizes=1
  Sum of Elements : Sum  Inputs=+
  Slct(C) : Outport
  wires:
  In(C)/1 -> Selector/1
  Selector/1 -> Sum of Elements/1
  Sum of Elements/1 -> Slct(C)/1

== system F3M_commonLib/Continuous MAPIT Recorder/TSS ==
  In(C) : Inport
  Enable : EnablePort
  MAPIT_OUT : ToWorkspace  VariableName=simout1  SaveFormat=Structure With Time  SampleTime=-1
  Squeeze : Squeeze
  wires:
  In(C)/1 -> Squeeze/1
  Squeeze/1 -> MAPIT_OUT/1

== system F3M_commonLib/Continuous to Discrete/Simulink Function ==
  Inport : Inport
  updateIsovec() : TriggerPort  TriggerType=function-call  IsSimulinkFunction=on  FunctionName=updateIsovec  FunctionVisibility=scoped  VariantControl=(inherit)
  y : ArgOut  DisableCoverage=on  PortDimensions=1677  ArgumentName=y
  wires:
  Inport/1 -> y/1

== system F3M_commonLib/Continuous to Discrete/Triggered Subsystem ==
  Inventory In : Inport
  In2 : Inport  Port=2
  Trigger : TriggerPort  VariantControl=(inherit)
  Inport : Outport
  Out2 : Outport  Port=2
  wires:
  Inventory In/1 -> Inport/1
  In2/1 -> Out2/1

== system F3M_commonLib/Custom Source Generator/Simulink Function ==
  getInitialIsos : TriggerPort  TriggerType=function-call  IsSimulinkFunction=on  FunctionName=getInitialIsos  FunctionVisibility=scoped  VariantControl=(inherit)
  Constant : Constant  Value=size
  Constant1 : Constant  Value=F3_ptableToArray(ptable,true)
  MATLAB Function : MATLAB Function  TreatAsAtomicUnit=on
  y : ArgOut  DisableCoverage=on  PortDimensions=1677  ArgumentName=y
  wires:
  MATLAB Function/1(y) -> y/1
  Constant/1 -> MATLAB Function/1(itemsize)
  Constant1/1 -> MATLAB Function/2(ptable)

== system F3M_commonLib/Discrete MAPIT Recorder/TSS ==
  readAttrib : TriggerPort  TriggerType=function-call  IsSimulinkFunction=on  FunctionName=readAttrib  FunctionVisibility=scoped  VariantControl=(inherit)
  MAPIT_OUT : ToWorkspace  VariableName=simout1  SaveFormat=Structure With Time  SampleTime=-1
  Selector : Selector  InputPortWidth=1677  IndexOptions=Index vector (dialog)  Indices=F3_getArrayPos(InString)  OutputSizes=1
  Sum of Elements : Sum  Inputs=+
  u : ArgIn  DisableCoverage=on  PortDimensions=1677  ArgumentName=u
  wires:
  Selector/1 -> Sum of Elements/1
  u/1 -> Selector/1
  Sum of Elements/1 -> MAPIT_OUT/1

== system F3M_commonLib/Discrete MAPIT Recorder/TSS1 ==
  readAttrib : TriggerPort  TriggerType=function-call  IsSimulinkFunction=on  FunctionName=readAttrib  FunctionVisibility=scoped  VariantControl=(inherit)
  MAPIT_OUT : ToWorkspace  VariableName=simout1  SaveFormat=Structure With Time  SampleTime=-1
  u : ArgIn  DisableCoverage=on  PortDimensions=1677  ArgumentName=u
  wires:
  u/1 -> MAPIT_OUT/1

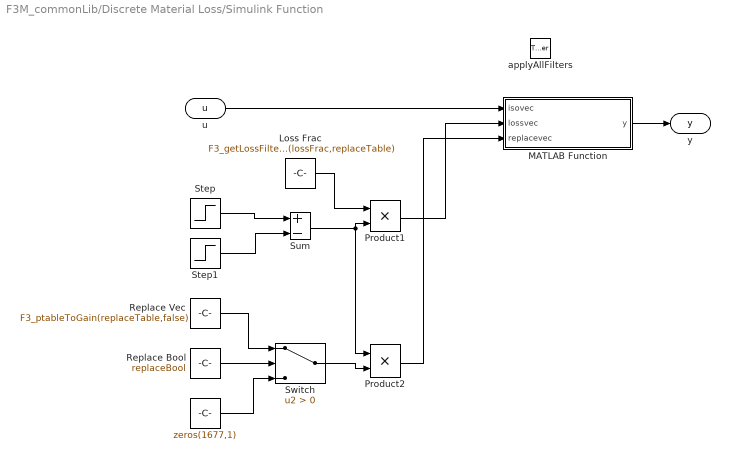
== system F3M_commonLib/Discrete Material Loss/Simulink Function ==
  applyAllFilters : TriggerPort  TriggerType=function-call  IsSimulinkFunction=on  FunctionName=applyAllFilters  FunctionVisibility=scoped  VariantControl=(inherit)
  " " : Constant  Value=zeros(1677,1)
  Loss Frac : Constant  Value=F3_getLossFilter(lossFrac,replaceTable)
  MATLAB Function : MATLAB Function  TreatAsAtomicUnit=on
  Product1 : Product
  Product2 : Product
  Replace Bool : Constant  Value=replaceBool
  Replace Vec : Constant  Value=F3_ptableToGain(replaceTable,false)
  Step : Step  Time=tStart
  Step1 : Step  Time=tEnd
  Sum : Sum  Inputs=+-
  Switch : Switch  Criteria=u2 > Threshold  SaturateOnIntegerOverflow=off  InputSameDT=off
  u : ArgIn  DisableCoverage=on  PortDimensions=1677  ArgumentName=u
  y : ArgOut  DisableCoverage=on  PortDimensions=1677  ArgumentName=y
  wires:
  u/1 -> MATLAB Function/1(isovec)
  Step/1 -> Sum/1
  Sum/1 -> Product1/2, Product2/1
  Loss Frac/1 -> Product1/1
  Replace Bool/1 -> Switch/2
  Replace Vec/1 -> Switch/1
  " "/1 -> Switch/3
  Switch/1 -> Product2/2
  Product1/1 -> MATLAB Function/2(lossvec)
  Product2/1 -> MATLAB Function/3(replacevec)
  MATLAB Function/1(y) -> y/1
  Step1/1 -> Sum/2

== system F3M_commonLib/Discrete Material Loss/Simulink Function1 ==
  updateCurrentEProperties : TriggerPort  TriggerType=function-call  IsSimulinkFunction=on  FunctionName=updateCurrentEProperties  FunctionVisibility=scoped  VariantControl=(inherit)
  u : ArgIn  DisableCoverage=on  PortDimensions=1677  ArgumentName=u
  Out1 : Outport
  wires:
  u/1 -> Out1/1

== system F3M_commonLib/Discrete Material Loss/Simulink Function2 ==
  u : Inport
  applyLossFilterLossE : TriggerPort  TriggerType=function-call  IsSimulinkFunction=on  FunctionName=applyLossFilterLossE  FunctionVisibility=scoped  VariantControl=(inherit)
  Loss Vec : Constant  Value=F3_getLossFilter(lossFrac,lossOverrideTab)
  MATLAB Function : MATLAB Function  TreatAsAtomicUnit=on
  Product1 : Product
  Step : Step  Time=tStart
  Step1 : Step  Time=tEnd
  Sum : Sum  Inputs=+-
  y : ArgOut  DisableCoverage=on  PortDimensions=1677  ArgumentName=y
  wires:
  u/1 -> MATLAB Function/1(isovec)
  MATLAB Function/1(y) -> y/1
  Step/1 -> Sum/1
  Product1/1 -> MATLAB Function/2(lossfrac)
  Loss Vec/1 -> Product1/1
  Step1/1 -> Sum/2
  Sum/1 -> Product1/2

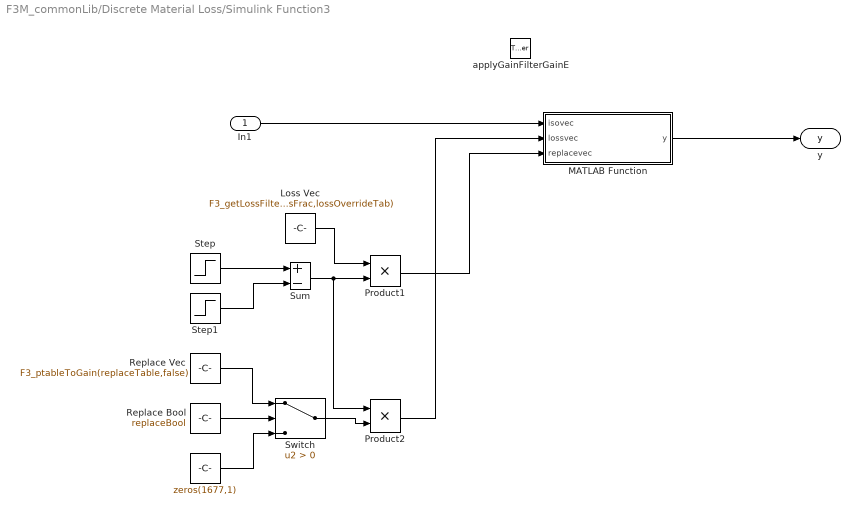
== system F3M_commonLib/Discrete Material Loss/Simulink Function3 ==
  In1 : Inport
  applyGainFilterGainE : TriggerPort  TriggerType=function-call  IsSimulinkFunction=on  FunctionName=applyGainFilterGainE  FunctionVisibility=scoped  VariantControl=(inherit)
  " " : Constant  Value=zeros(1677,1)
  Loss Vec : Constant  Value=F3_getLossFilter(lossFrac,lossOverrideTab)
  MATLAB Function : MATLAB Function  TreatAsAtomicUnit=on
  Product1 : Product
  Product2 : Product
  Replace Bool : Constant  Value=replaceBool
  Replace Vec : Constant  Value=F3_ptableToGain(replaceTable,false)
  Step : Step  Time=tStart
  Step1 : Step  Time=tEnd
  Sum : Sum  Inputs=+-
  Switch : Switch  Criteria=u2 > Threshold  SaturateOnIntegerOverflow=off  InputSameDT=off
  y : ArgOut  DisableCoverage=on  PortDimensions=1677  ArgumentName=y
  wires:
  In1/1 -> MATLAB Function/1(isovec)
  MATLAB Function/1(y) -> y/1
  Sum/1 -> Product2/1, Product1/2
  Step/1 -> Sum/1
  Product1/1 -> MATLAB Function/3(replacevec)
  Product2/1 -> MATLAB Function/2(lossvec)
  Switch/1 -> Product2/2
  Loss Vec/1 -> Product1/1
  Step1/1 -> Sum/2
  " "/1 -> Switch/3
  Replace Bool/1 -> Switch/2
  Replace Vec/1 -> Switch/1

== system F3M_commonLib/Discrete to Continuous/Simulink Function ==
  Inport : Inport
  getIsoVec : TriggerPort  TriggerType=function-call  IsSimulinkFunction=on  FunctionName=getIsoVec  FunctionVisibility=scoped  VariantControl=(inherit)
  MATLAB Function : MATLAB Function  TreatAsAtomicUnit=on
  u : ArgIn  DisableCoverage=on  PortDimensions=1677  ArgumentName=u
  Out1 : Outport
  Out2 : Outport  Port=2
  wires:
  Inport/1 -> Out2/1
  u/1 -> MATLAB Function/1(isovec)
  MATLAB Function/1(y) -> Out1/1

== system F3M_commonLib/Entity Hold (Periodic)/Simulink Function ==
  updateInv : TriggerPort  TriggerType=function-call  IsSimulinkFunction=on  FunctionName=updateInv  FunctionVisibility=scoped  VariantControl=(inherit)
  MATLAB Function : MATLAB Function  TreatAsAtomicUnit=on
  isovec : ArgIn  DisableCoverage=on  PortDimensions=1677  ArgumentName=isovec
  utype : ArgIn  DisableCoverage=on  Port=2  ArgumentName=utype
  y : Outport
  wires:
  utype/1 -> MATLAB Function/2(utype)
  MATLAB Function/1(y) -> y/1
  isovec/1 -> MATLAB Function/1(isovec)

== system F3M_commonLib/Entity Process and Hold/Simulink Function ==
  calculateNewEntity : TriggerPort  TriggerType=function-call  IsSimulinkFunction=on  FunctionName=calculateNewEntity  FunctionVisibility=scoped  VariantControl=(inherit)
  Constant : Constant  Value=F3_ptableToArray(ptable,false)
  MATLAB Function : MATLAB Function  TreatAsAtomicUnit=on
  isovec : ArgIn  DisableCoverage=on  PortDimensions=1677  ArgumentName=isovec
  etype : ArgIn  DisableCoverage=on  Port=2  ArgumentName=etype
  mod_entity : ArgOut  DisableCoverage=on  PortDimensions=1677  ArgumentName=mod_entity
  wires:
  MATLAB Function/1(mod_entity) -> mod_entity/1
  etype/1 -> MATLAB Function/3(etype)
  Constant/1 -> MATLAB Function/2(ptable_array)
  isovec/1 -> MATLAB Function/1(isovec)

== system F3M_commonLib/Entity Process and Hold/Simulink Function2 ==
  updateLatestEntity : TriggerPort  TriggerType=function-call  IsSimulinkFunction=on  FunctionName=updateLatestEntity  FunctionVisibility=scoped  VariantControl=(inherit)
  u : ArgIn  DisableCoverage=on  PortDimensions=1677  ArgumentName=u
  Out1 : Outport
  wires:
  u/1 -> Out1/1

== system F3M_commonLib/Entity Process and Hold/Simulink Function3 ==
  In1 : Inport
  getEntityValue : TriggerPort  TriggerType=function-call  IsSimulinkFunction=on  FunctionName=getEntityValue  FunctionVisibility=scoped  VariantControl=(inherit)
  y : ArgOut  DisableCoverage=on  PortDimensions=1677  ArgumentName=y
  wires:
  In1/1 -> y/1

== system F3M_commonLib/Entity Process and Hold/Subsystem ==
  updateInv : TriggerPort  TriggerType=function-call  IsSimulinkFunction=on  FunctionName=updateInv  FunctionVisibility=scoped  VariantControl=(inherit)
  MATLAB Function : MATLAB Function  TreatAsAtomicUnit=on
  isovec : ArgIn  DisableCoverage=on  PortDimensions=1677  ArgumentName=isovec
  utype : ArgIn  DisableCoverage=on  Port=2  ArgumentName=utype
  y : Outport
  wires:
  isovec/1 -> MATLAB Function/1(isovec)
  MATLAB Function/1(y) -> y/1
  utype/1 -> MATLAB Function/2(utype)
